simulink model "VelocityModel"  (R2018b)
settings: Solver=VariableStepAuto  StartTime=0.0  StopTime=1000.0  RelTol=1e-3
values from neighbouring files (symbols this model uses):
  Adisc = sysd.A    [Constants.m]
  Bdisc = sysd.B    [Constants.m]
  thetaR = 0    [Constants.m]
undefined symbols (not defined in the file or in its folder): K
libraries: dspinverses x1
settings Model: Creator=simarkareer  LastModifiedBy=simarkareer

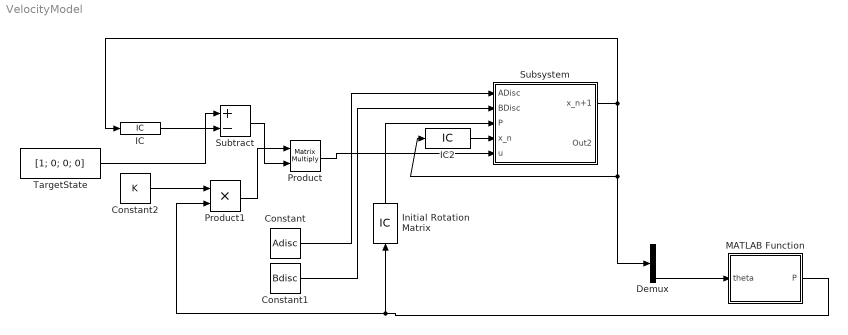
== system VelocityModel ==
  Constant : Constant  Value=Adisc
  Constant1 : Constant  Value=Bdisc
  Constant2 : Constant  Value=K  VectorParams1D=off
  Demux : Demux
  IC : InitialCondition  Value=[0; 0; 0; 0]
  IC2 : InitialCondition  Value=[0; 0; 0; 0]
  "Initial Rotation Matrix " : InitialCondition  Value=[cos(thetaR) -sin(thetaR) 0 0; sin(thetaR) cos(thetaR) 0 0; 0 0 1 0; 0 0 0 1]
  MATLAB Function : MATLAB Function  TreatAsAtomicUnit=on
  Product : Product  Multiplication=Matrix(*)
  Product1 : Product
  Subsystem : Subsystem
  Subtract : Sum  Inputs=+-
  "TargetState " : Constant  Value=[1; 0; 0; 0]  VectorParams1D=off
  wires:
  Constant/1 -> Subsystem/1(ADisc)
  Subsystem/1(x_n+1) -> IC2/1, Demux/1, IC/1
  Demux/4 -> MATLAB Function/1(theta)
  Constant2/1 -> Product1/1
  Constant1/1 -> Subsystem/2(BDisc)
  Product/1 -> Subsystem/5("u ")
  MATLAB Function/1(P) -> Product1/2, "Initial Rotation Matrix "/1
  IC/1 -> Subtract/2
  "TargetState "/1 -> Subtract/1
  Product1/1 -> Product/1
  Subtract/1 -> Product/2
  IC2/1 -> Subsystem/4(x_n)
  "Initial Rotation Matrix "/1 -> Subsystem/3(P)

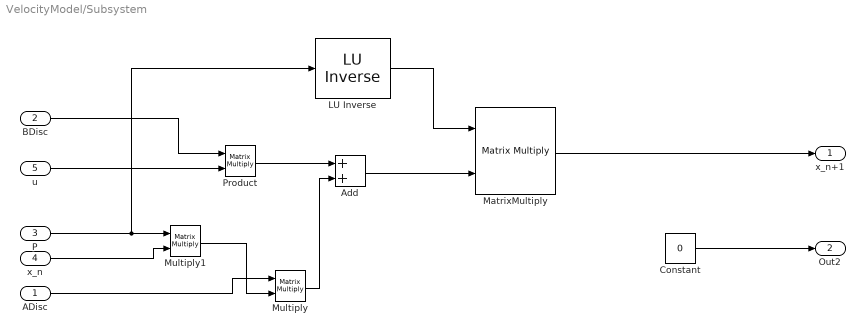
== system VelocityModel/Subsystem ==
  ADisc : Inport
  BDisc : Inport  Port=2
  P : Inport  Port=3
  x_n : Inport  Port=4
  "u " : Inport  Port=5
  " LU Inverse" : dspinverses/ LU Inverse
      settings: SourceProductName=DSP System Toolbox
  Add : Sum
  Constant : Constant  Value=0
  MatrixMultiply : Product  Multiplication=Matrix(*)
  Multiply : Product  Multiplication=Matrix(*)
  Multiply1 : Product  Multiplication=Matrix(*)
  Product : Product  Multiplication=Matrix(*)
  x_n+1 : Outport
  Out2 : Outport  Port=2
  wires:
  P/1 -> Multiply1/1, " LU Inverse"/1
  x_n/1 -> Multiply1/2
  Product/1 -> Add/1
  Multiply/1 -> Add/2
  Add/1 -> MatrixMultiply/2
  MatrixMultiply/1 -> x_n+1/1
  Constant/1 -> Out2/1
  " LU Inverse"/1 -> MatrixMultiply/1
  BDisc/1 -> Product/1
  "u "/1 -> Product/2
  Multiply1/1 -> Multiply/2
  ADisc/1 -> Multiply/1

== matlab function VelocityModel/MATLAB Function ==
  data: theta input; P output
function P = RotationM(theta)
P = [
    cos(theta), -sin(theta), 0, 0;
    sin(theta), cos(theta), 0, 0;
    0, 0, 1, 0;
    0, 0, 0, 1;
];
